simulink model "Rint_model_decibel"  (R2023b)
settings: Solver=VariableStepAuto  StartTime=0.0  StopTime=3600  RelTol=1e-3
values from neighbouring files (symbols this model uses):
  A_cell = cell_length*cell_width    (= 0.051302)    [Rint_script_decibel.m]
  Cp_cell = 810.5328    [Rint_script_decibel.m]
  h_cell = 5    [Rint_script_decibel.m]
  m_cell = 0.72    [Rint_script_decibel.m]
  OCV_LUT = [3.49; 3.55; 3.62; 3.71; 3.91; 4.17; 4.19]    [Rint_script_decibel.m]
  R_int_LUT = [0.0085; 0.0085; 0.0087; 0.0082; 0.0083; 0.0085; 0.0097]    [Rint_script_decibel.m]
  SOC_LUT = [0; 0.1; 0.25; 0.5; 0.75; 0.9; 1.0]    [Rint_script_decibel.m]
  T_amb = 293.15    [Rint_script_decibel.m]
settings Model: Creator=deepp  LastModifiedBy=deepp

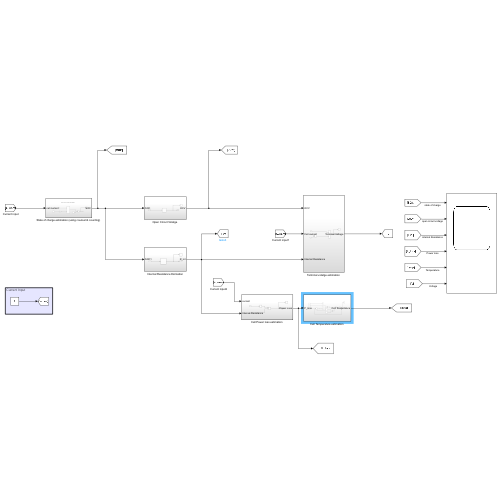
[thumbnail: Simulink's stored preview of the top-level diagram]
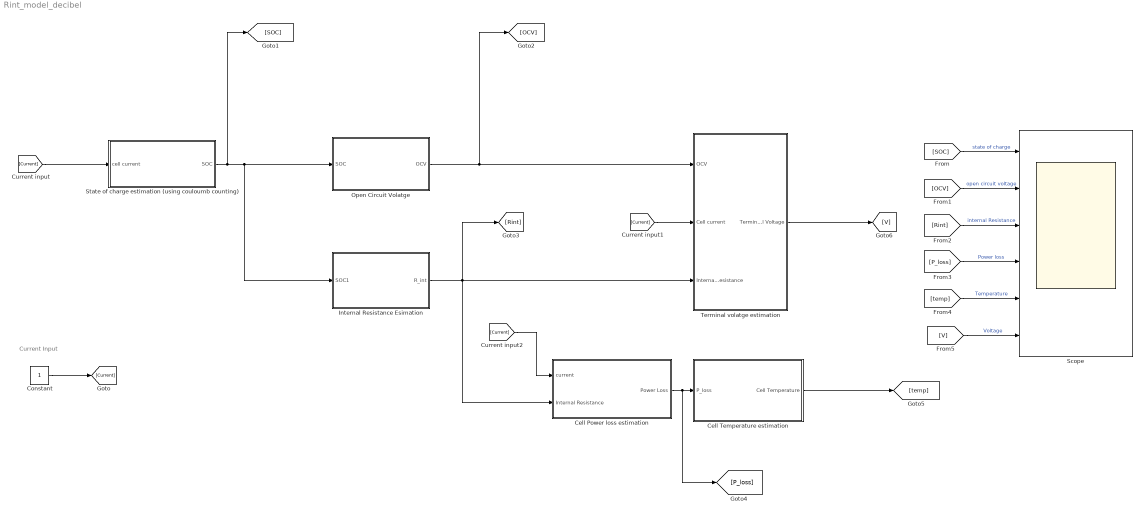
== system Rint_model_decibel ==
  note: Current Input
  "Cell Power loss estimation " : Subsystem
  "Cell Temperature estimation " : Subsystem
  Constant : Constant
  Internal Resistance Esimation : Subsystem
  "Open Circuit Volatge " : Subsystem
  Scope : Scope  NumInputPorts=6
  "State of charge estimation (using couloumb counting) " : Subsystem
  "Terminal volatge estimation " : Subsystem
  wires:
  "State of charge estimation (using couloumb counting) "/1(SOC) -> [SOC], Internal Resistance Esimation/1(SOC1), "Open Circuit Volatge "/1(SOC)
  "Open Circuit Volatge "/1(OCV) -> [OCV], "Terminal volatge estimation "/1(OCV)
  Internal Resistance Esimation/1(R_int) -> [Rint], "Cell Power loss estimation "/2("Internal Resistance "), "Terminal volatge estimation "/3(Internal Resistance)
  "Cell Power loss estimation "/1(Power Loss) -> [P_loss], "Cell Temperature estimation "/1(P_loss)
  Constant/1 -> [Current]
  [Current] -> "State of charge estimation (using couloumb counting) "/1(cell current)
  [Current] -> "Terminal volatge estimation "/2(Cell current)
  [Current] -> "Cell Power loss estimation "/1(current)
  "Cell Temperature estimation "/1(Cell Temperature) -> [temp]
  "Terminal volatge estimation "/1(Terminal Voltage) -> [V]
  [SOC] -> Scope/1  "state of charge"
  [OCV] -> Scope/2  "open circuit voltage"
  [Rint] -> Scope/3  "internal Resistance"
  [P_loss] -> Scope/4  "Power loss"
  [temp] -> Scope/5  "Temperature"
  [V] -> Scope/6  "Voltage"

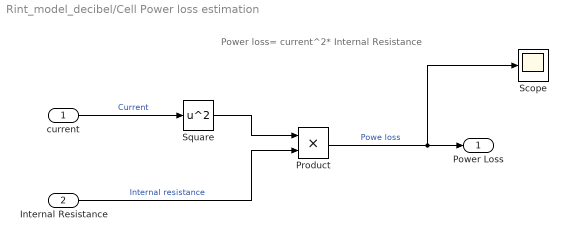
== system Rint_model_decibel/Cell Power loss estimation  ==
  note: Power loss= current^2* Internal Resistance
  current : Inport
  "Internal Resistance " : Inport  Port=2
  Product : Product
  Scope : Scope
  Square : Math  Operator=square
  Power Loss : Outport
  wires:
  current/1 -> Square/1  "Current"
  Square/1 -> Product/1
  "Internal Resistance "/1 -> Product/2  "Internal resistance"
  Product/1 -> Scope/1, Power Loss/1  "Powe loss"

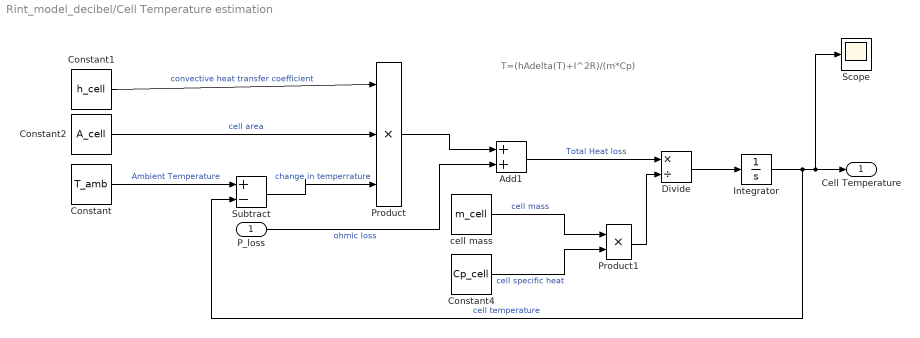
== system Rint_model_decibel/Cell Temperature estimation  ==
  note: T=(hAdelta(T)+I^2R)/(m*Cp)
  P_loss : Inport
  Add1 : Sum
  Constant : Constant  Value=T_amb
  Constant1 : Constant  Value=h_cell
  Constant2 : Constant  Value=A_cell
  Constant4 : Constant  Value=Cp_cell
  Divide : Product  Inputs=*/
  Integrator : Integrator  InitialCondition=T_amb
  Product : Product  Inputs=3
  Product1 : Product
  Scope : Scope
  Subtract : Sum  Inputs=+-
  cell mass : Constant  Value=m_cell
  Cell Temperature : Outport
  wires:
  Constant1/1 -> Product/1  "convective heat transfer coefficient"
  Constant2/1 -> Product/2  "cell area"
  Constant/1 -> Subtract/1  "Ambient Temperature"
  Subtract/1 -> Product/3  "change in temperrature"
  Product/1 -> Add1/1
  Add1/1 -> Divide/1  "Total Heat loss"
  P_loss/1 -> Add1/2  "ohmic loss"
  cell mass/1 -> Product1/1  "cell mass"
  Constant4/1 -> Product1/2  "cell specific heat"
  Product1/1 -> Divide/2
  Divide/1 -> Integrator/1
  Integrator/1 -> Subtract/2, Scope/1, Cell Temperature/1  "cell temperature"

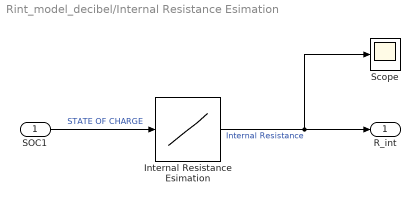
== system Rint_model_decibel/Internal Resistance Esimation ==
  SOC1 : Inport
  "Internal Resistance Esimation " : Lookup_n-D  NumberOfTableDimensions=1  BreakpointsForDimension1=SOC_LUT  Table=R_int_LUT  InternalRulePriority=Speed  RndMeth=Simplest
  Scope : Scope
  R_int : Outport
  wires:
  SOC1/1 -> "Internal Resistance Esimation "/1  "STATE OF CHARGE"
  "Internal Resistance Esimation "/1 -> Scope/1, R_int/1  "Internal Resistance"

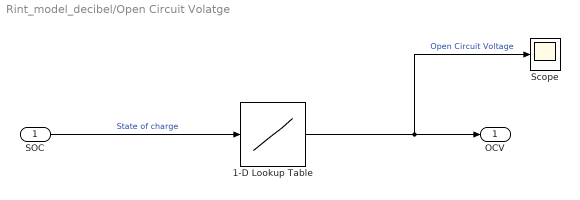
== system Rint_model_decibel/Open Circuit Volatge  ==
  SOC : Inport
  1-D Lookup Table : Lookup_n-D  NumberOfTableDimensions=1  BreakpointsForDimension1=SOC_LUT  Table=OCV_LUT  InternalRulePriority=Speed  RndMeth=Simplest
  Scope : Scope
  OCV : Outport
  wires:
  SOC/1 -> 1-D Lookup Table/1  "State of charge"
  1-D Lookup Table/1 -> Scope/1, OCV/1  "Open Circuit Voltage"

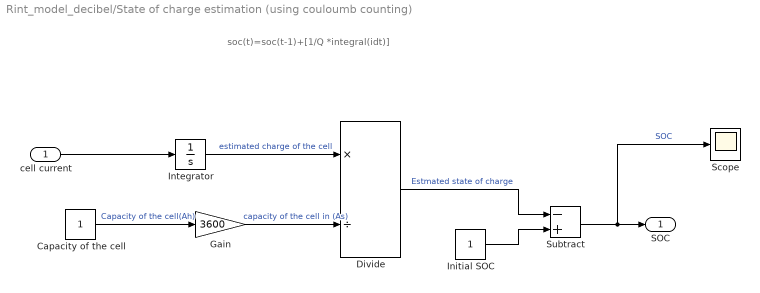
== system Rint_model_decibel/State of charge estimation (using couloumb counting)  ==
  note: soc(t)=soc(t-1)+[1/Q *integral(idt)]
  cell current : Inport
  Capacity of the cell : Constant
  Divide : Product  Inputs=*/
  Gain : Gain  Gain=3600
  Initial SOC : Constant
  Integrator : Integrator
  Scope : Scope
  Subtract : Sum  Inputs=-+
  SOC : Outport
  wires:
  cell current/1 -> Integrator/1
  Integrator/1 -> Divide/1  "estimated charge of the cell"
  Capacity of the cell/1 -> Gain/1  "Capacity of the cell(Ah)"
  Initial SOC/1 -> Subtract/2
  Subtract/1 -> Scope/1, SOC/1  "SOC"
  Divide/1 -> Subtract/1  "Estmated state of charge"
  Gain/1 -> Divide/2  "capacity of the cell in (As)"

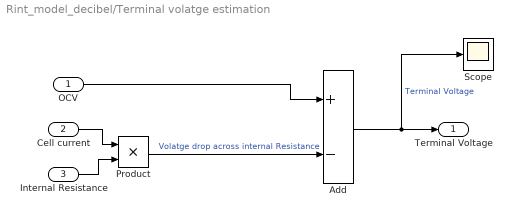
== system Rint_model_decibel/Terminal volatge estimation  ==
  OCV : Inport
  Cell current : Inport  Port=2
  Internal Resistance : Inport  Port=3
  Add : Sum  Inputs=+-
  Product : Product
  Scope : Scope
  Terminal Voltage : Outport
  wires:
  OCV/1 -> Add/1
  Add/1 -> Scope/1, Terminal Voltage/1  "Terminal Voltage"
  Cell current/1 -> Product/1
  Internal Resistance/1 -> Product/2
  Product/1 -> Add/2  "Volatge drop across internal Resistance"
